simulink model "chris_3R_hsv_all_primitives_sinking_vortex"  (R2024b)
settings: Solver=FixedStepDiscrete  StartTime=0.0  StopTime=30  FixedStep=0.1  MaxStep=0.1  RelTol=1e-3
libraries: neural x110, realtime_pacer_lib x1, simulink x1
(part 6 of 7)

== system chris_3R_hsv_all_primitives_sinking_vortex/tidal_hsv_tuning1/RGB to hue_sat for_celeste/celeste_sat_net/Layer 2/LW{2,1} ==
  "ad{2,1}" : Inport  PortDimensions=6
      mask Display: e = 0.06;c1 = [120 230 180]/255;c2 = ([120 230 180]+0)/(256+128);c3 = ([120 230 180]+128)/(256+128);patch([0 1 1 0],[0 0 1 1],c1);patch([0 1 1 1-e 1-e 0+e],[0 0 1 1-e 0+e 0+e],c2);patch([0 0 1 1-e 0+e 0+e],[0 1 1 1-e 1-e 0+e],c3);plot([0 1 1 0 0],[0 0 1 1 0]);
  "IW{2,1}(1,:)'" : Constant  Value=[1.2757889938032482834984193686977960169315338134765625;-0.7126078429664080005068171885795891284942626953125;-2.413344046511821883171933222911320626735687255859375;-1.458997927672031291734811020432971417903900146484375;-0.83989823818357633999909239719272591173648834228515625;1.7854337780265587820593964352156035602092742919921875]
      mask Display: e = 0.06;c1 = [120 150 230]/255;c2 = ([120 150 230]+0)/383;c3 = ([120 150 230]+128)/383;patch([0 1 1 0],[0 0 1 1],c1);patch([0 1 1 1-e 1-e 0+e],[0 0 1 1-e 0+e 0+e],c2);patch([0 0 1 1-e 0+e 0+e],[0 1 1 1-e 1-e 0+e],c3);plot([0 1 1 0 0],[0 0 1 1 0]);disp('weights');
  "IW{2,1}(2,:)'" : Constant  Value=[-1.6571971168098029725257447353214956820011138916015625;-0.67977626560509663011799830201198346912860870361328125;0.51865396369048488711683830842957831919193267822265625;0.243374659103428425677151381023577414453029632568359375;-0.076285515094898281862612066106521524488925933837890625;1.29330601294184877048110138275660574436187744140625]
      mask Display: e = 0.06;c1 = [120 150 230]/255;c2 = ([120 150 230]+0)/383;c3 = ([120 150 230]+128)/383;patch([0 1 1 0],[0 0 1 1],c1);patch([0 1 1 1-e 1-e 0+e],[0 0 1 1-e 0+e 0+e],c2);patch([0 0 1 1-e 0+e 0+e],[0 1 1 1-e 1-e 0+e],c3);plot([0 1 1 0 0],[0 0 1 1 0]);disp('weights');
  "IW{2,1}(3,:)'" : Constant  Value=[1.377295451076403054457841790281236171722412109375;0.01268764281998376909632586517773233936168253421783447265625;0.0289104963224421605827441084102247259579598903656005859375;-1.145112921630900615355130867101252079010009765625;-1.1470518023551152797523400295176543295383453369140625;0.7180170108229269043675913053448311984539031982421875]
      mask Display: e = 0.06;c1 = [120 150 230]/255;c2 = ([120 150 230]+0)/383;c3 = ([120 150 230]+128)/383;patch([0 1 1 0],[0 0 1 1],c1);patch([0 1 1 1-e 1-e 0+e],[0 0 1 1-e 0+e 0+e],c2);patch([0 0 1 1-e 0+e 0+e],[0 1 1 1-e 1-e 0+e],c3);plot([0 1 1 0 0],[0 0 1 1 0]);disp('weights');
  "IW{2,1}(4,:)'" : Constant  Value=[-0.50505648910016531782929405380855314433574676513671875;1.641889229081123335873826363240368664264678955078125;0.36309788129570963466363764382549561560153961181640625;2.063260495572241115525002896902151405811309814453125;-1.3457901837695616098500295265694148838520050048828125;3.00694287438520913013917379430495202541351318359375]
      mask Display: e = 0.06;c1 = [120 150 230]/255;c2 = ([120 150 230]+0)/383;c3 = ([120 150 230]+128)/383;patch([0 1 1 0],[0 0 1 1],c1);patch([0 1 1 1-e 1-e 0+e],[0 0 1 1-e 0+e 0+e],c2);patch([0 0 1 1-e 0+e 0+e],[0 1 1 1-e 1-e 0+e],c3);plot([0 1 1 0 0],[0 0 1 1 0]);disp('weights');
  "IW{2,1}(5,:)'" : Constant  Value=[1.747547092995427764350324650877155363559722900390625;1.21424683147417855622052229591645300388336181640625;-2.265290257368467674581324899918399751186370849609375;-0.38255863058397288067880026574130170047283172607421875;1.7408214945567326292774623652803711593151092529296875;-1.030400253471217109080271256971172988414764404296875]
      mask Display: e = 0.06;c1 = [120 150 230]/255;c2 = ([120 150 230]+0)/383;c3 = ([120 150 230]+128)/383;patch([0 1 1 0],[0 0 1 1],c1);patch([0 1 1 1-e 1-e 0+e],[0 0 1 1-e 0+e 0+e],c2);patch([0 0 1 1-e 0+e 0+e],[0 1 1 1-e 1-e 0+e],c3);plot([0 1 1 0 0],[0 0 1 1 0]);disp('weights');
  Mux : Mux  Inputs=5
      mask Display: e = 0.06;c1 = [120 150 230]/255;c2 = ([120 150 230]+0)/383;c3 = ([120 150 230]+128)/383;patch([0 1 1 0],[0 0 1 1],c1);patch([0 1 1 1-e 1-e 0+e],[0 0 1 1-e 0+e 0+e],c2);patch([0 0 1 1-e 0+e 0+e],[0 1 1 1-e 1-e 0+e],c3);plot([0 1 1 0 0],[0 0 1 1 0]);disp('Mux');
  dotprod{1..5} (5 alike) : neural/Weight Functions/dotprod
  "lz{2,1}" : Outport
      mask Display: e = 0.06;c1 = [120 230 180]/255;c2 = ([120 230 180]+0)/(256+128);c3 = ([120 230 180]+128)/(256+128);patch([0 1 1 0],[0 0 1 1],c1);patch([0 1 1 1-e 1-e 0+e],[0 0 1 1-e 0+e 0+e],c2);patch([0 0 1 1-e 0+e 0+e],[0 1 1 1-e 1-e 0+e],c3);plot([0 1 1 0 0],[0 0 1 1 0]);
  wires:
  "IW{2,1}(1,:)'"/1 -> dotprod1/1
  "ad{2,1}"/1 -> dotprod1/2, dotprod2/2, dotprod3/2, dotprod4/2, dotprod5/2
  dotprod1/1 -> Mux/1
  "IW{2,1}(2,:)'"/1 -> dotprod2/1
  dotprod2/1 -> Mux/2
  "IW{2,1}(3,:)'"/1 -> dotprod3/1
  dotprod3/1 -> Mux/3
  "IW{2,1}(4,:)'"/1 -> dotprod4/1
  dotprod4/1 -> Mux/4
  "IW{2,1}(5,:)'"/1 -> dotprod5/1
  dotprod5/1 -> Mux/5
  Mux/1 -> "lz{2,1}"/1

== system chris_3R_hsv_all_primitives_sinking_vortex/tidal_hsv_tuning1/RGB to hue_sat for_celeste/celeste_sat_net/Layer 3/Delays 1 ==
  "p{3}" : Inport  PortDimensions=5
      mask Display: e = 0.06;c1 = [120 230 180]/255;c2 = ([120 230 180]+0)/(256+128);c3 = ([120 230 180]+128)/(256+128);patch([0 1 1 0],[0 0 1 1],c1);patch([0 1 1 1-e 1-e 0+e],[0 0 1 1-e 0+e 0+e],c2);patch([0 0 1 1-e 0+e 0+e],[0 1 1 1-e 1-e 0+e],c3);plot([0 1 1 0 0],[0 0 1 1 0]);
  mux : Mux  Inputs=1
      mask Display: e = 0.06;c1 = [120 150 230]/255;c2 = ([120 150 230]+0)/383;c3 = ([120 150 230]+128)/383;patch([0 1 1 0],[0 0 1 1],c1);patch([0 1 1 1-e 1-e 0+e],[0 0 1 1-e 0+e 0+e],c2);patch([0 0 1 1-e 0+e 0+e],[0 1 1 1-e 1-e 0+e],c3);plot([0 1 1 0 0],[0 0 1 1 0]);disp('Mux')
  "pd{3,2}" : Outport
      mask Display: e = 0.06;c1 = [120 230 180]/255;c2 = ([120 230 180]+0)/(256+128);c3 = ([120 230 180]+128)/(256+128);patch([0 1 1 0],[0 0 1 1],c1);patch([0 1 1 1-e 1-e 0+e],[0 0 1 1-e 0+e 0+e],c2);patch([0 0 1 1-e 0+e 0+e],[0 1 1 1-e 1-e 0+e],c3);plot([0 1 1 0 0],[0 0 1 1 0]);
  wires:
  "p{3}"/1 -> mux/1
  mux/1 -> "pd{3,2}"/1

== system chris_3R_hsv_all_primitives_sinking_vortex/tidal_hsv_tuning1/RGB to hue_sat for_celeste/celeste_sat_net/Layer 3/LW{3,2} ==
  "ad{3,2}" : Inport  PortDimensions=5
      mask Display: e = 0.06;c1 = [120 230 180]/255;c2 = ([120 230 180]+0)/(256+128);c3 = ([120 230 180]+128)/(256+128);patch([0 1 1 0],[0 0 1 1],c1);patch([0 1 1 1-e 1-e 0+e],[0 0 1 1-e 0+e 0+e],c2);patch([0 0 1 1-e 0+e 0+e],[0 1 1 1-e 1-e 0+e],c3);plot([0 1 1 0 0],[0 0 1 1 0]);
  "IW{3,2}(1,:)'" : Constant  Value=[-2.69284198651846651273444877006113529205322265625;1.3716092909789459053371274421806447207927703857421875;2.600820941170569167155690593062900006771087646484375;1.14691405759365405714333974174223840236663818359375;-1.59834977518721199629680995712988078594207763671875]
      mask Display: e = 0.06;c1 = [120 150 230]/255;c2 = ([120 150 230]+0)/383;c3 = ([120 150 230]+128)/383;patch([0 1 1 0],[0 0 1 1],c1);patch([0 1 1 1-e 1-e 0+e],[0 0 1 1-e 0+e 0+e],c2);patch([0 0 1 1-e 0+e 0+e],[0 1 1 1-e 1-e 0+e],c3);plot([0 1 1 0 0],[0 0 1 1 0]);disp('weights');
  Mux : Mux  Inputs=1
      mask Display: e = 0.06;c1 = [120 150 230]/255;c2 = ([120 150 230]+0)/383;c3 = ([120 150 230]+128)/383;patch([0 1 1 0],[0 0 1 1],c1);patch([0 1 1 1-e 1-e 0+e],[0 0 1 1-e 0+e 0+e],c2);patch([0 0 1 1-e 0+e 0+e],[0 1 1 1-e 1-e 0+e],c3);plot([0 1 1 0 0],[0 0 1 1 0]);disp('Mux');
  dotprod1 : neural/Weight Functions/dotprod
  "lz{3,2}" : Outport
      mask Display: e = 0.06;c1 = [120 230 180]/255;c2 = ([120 230 180]+0)/(256+128);c3 = ([120 230 180]+128)/(256+128);patch([0 1 1 0],[0 0 1 1],c1);patch([0 1 1 1-e 1-e 0+e],[0 0 1 1-e 0+e 0+e],c2);patch([0 0 1 1-e 0+e 0+e],[0 1 1 1-e 1-e 0+e],c3);plot([0 1 1 0 0],[0 0 1 1 0]);
  wires:
  "IW{3,2}(1,:)'"/1 -> dotprod1/1
  "ad{3,2}"/1 -> dotprod1/2
  dotprod1/1 -> Mux/1
  Mux/1 -> "lz{3,2}"/1

== matlab function chris_3R_hsv_all_primitives_sinking_vortex/Cluster_Controller_HSV_average_direction_and_mag_follower/Cluster Velocities to Cartesian Velocities ==
  data: fwdkin input; xc_err input; x1 output; zc_err input; thC_err input; a_err input; b_err input; C_err input; z1 output; th1 output; x2 output; z2 output; th2 output; x3 output; z3 output; th3 output
function [x1, z1,th1, x2,z2,th2, x3,z3, th3] = InverseJabobian(fwdkin, xc_err, zc_err, thC_err, a_err, b_err, C_err)
%% Unpacking the information from fwd_kin
p = fwdkin(1);
q = fwdkin(2);
beta = fwdkin(3);
xc = fwdkin(4);
yc = fwdkin(5);
theta_c = fwdkin(6);
yc_err = zc_err;
theta_c_err = thC_err;
p_err = a_err;
q_err = b_err;
beta_err = C_err;
%% Inverse Kinematics
  % Calculate x1, y1, and theta1 (Equations 12, 13, and 14)
r = sqrt((q + p*cos(beta))^2 + (p*sin(beta))^2);
  
x1 = xc + (1/3)*r*sin(theta_c);
y1 = yc + (1/3)*r*cos(theta_c);
%theta1 = phi1 - theta_c;
% Calculate x2, y2, and theta2 (Equations 15, 16, and 17)
x2 = xc + (1/3)*r*sin(theta_c) - p*sin(beta/2 + theta_c);
y2 = yc + (1/3)*r*cos(theta_c) - p*cos(beta/2 + theta_c);
%theta2 = phi2 - theta_c;
% Calculate x3, y3, and theta3 (Equations 18, 19, and 20)
x3 = xc + (1/3)*r*sin(theta_c) + q*sin(beta/2 - theta_c);
y3 = yc + (1/3)*r*cos(theta_c) - q*cos(beta/2 - theta_c);
%theta3 = phi3 - theta_c;
%% Now to take the partial derivates
% syms p q beta xc yc theta_c p_err q_err beta_err xc_err yc_err theta_c_err
% 
% % Define the equations
% eqs = [
%   xc + (1/3)*(sqrt((q + p*cos(beta))^2 + (p*sin(beta))^2))*sin(theta_c); % x1
%   yc + (1/3)*(sqrt((q + p*cos(beta))^2 + (p*sin(beta))^2))*cos(theta_c); % y1
%   xc + (1/3)*(sqrt((q + p*cos(beta))^2 + (p*sin(beta))^2))*sin(theta_c) - p*sin(beta/2 + theta_c); % x2
%   yc + (1/3)*(sqrt((q + p*cos(beta))^2 + (p*sin(beta))^2))*cos(theta_c) - p*cos(beta/2 + theta_c); % y2
%   xc + (1/3)*(sqrt((q + p*cos(beta))^2 + (p*sin(beta))^2))*sin(theta_c) + q*sin(beta/2 - theta_c); % x3
%   yc + (1/3)*(sqrt((q + p*cos(beta))^2 + (p*sin(beta))^2))*cos(theta_c) - q*cos(beta/2 - theta_c)  % y3
% ];
% 
% % Define the variables for differentiation
% vars = [p, q, beta, xc, yc, theta_c];
% 
% % Define the errors
% errs = [p_err, q_err, beta_err, xc_err, yc_err, theta_c_err];
% 
% % Initialize an array to store the sums (as symbolic)
% sums = sym(zeros(length(eqs), 1));
% 
% % Loop through equations and variables
% for i = 1:length(eqs)
%   for j = 1:length(vars)
%     derivative = diff(eqs(i), vars(j));
%     sums(i) = sums(i) + derivative * errs(j);
%   end
% end
% 
% % Display the results
% disp(simplify(sums(1)))
% disp(simplify(sums(2)))
% disp(simplify(sums(3)))
% disp(simplify(sums(4)))
% disp(simplify(sums(5)))
% disp(simplify(sums(6)))
%% Now to sum it all up
x1 =(3*xc_err*(p^2 + 2*cos(beta)*p*q + q^2)^(1/2) + p*p_err*sin(theta_c) + q*q_err*sin(theta_c) + p^2*theta_c_err*cos(theta_c) + q^2*theta_c_err*cos(theta_c) + p*q_err*cos(beta)*sin(theta_c) + p_err*q*cos(beta)*sin(theta_c) + 2*p*q*theta_c_err*cos(beta)*cos(theta_c) - beta_err*p*q*sin(beta)*sin(theta_c))/(3*(p^2 + 2*cos(beta)*p*q + q^2)^(1/2));
 
z1 = (3*yc_err*(p^2 + 2*cos(beta)*p*q + q^2)^(1/2) + p*p_err*cos(theta_c) + q*q_err*cos(theta_c) - p^2*theta_c_err*sin(theta_c) - q^2*theta_c_err*sin(theta_c) + p*q_err*cos(beta)*cos(theta_c) + p_err*q*cos(beta)*cos(theta_c) - beta_err*p*q*sin(beta)*cos(theta_c) - 2*p*q*theta_c_err*cos(beta)*sin(theta_c))/(3*(p^2 + 2*cos(beta)*p*q + q^2)^(1/2));
 
x2 = xc_err - p_err*(sin(beta/2 + theta_c) - (sin(theta_c)*(p + q*cos(beta)))/(3*(p^2 + 2*cos(beta)*p*q + q^2)^(1/2))) - beta_err*((p*cos(beta/2 + theta_c))/2 + (p*q*sin(beta)*sin(theta_c))/(3*(p^2 + 2*cos(beta)*p*q + q^2)^(1/2))) + theta_c_err*((cos(theta_c)*(p^2 + 2*cos(beta)*p*q + q^2)^(1/2))/3 - p*cos(beta/2 + theta_c)) + (q_err*sin(theta_c)*(q + p*cos(beta)))/(3*(p^2 + 2*cos(beta)*p*q + q^2)^(1/2));
 
z2 = yc_err - p_err*(cos(beta/2 + theta_c) - (cos(theta_c)*(p + q*cos(beta)))/(3*(p^2 + 2*cos(beta)*p*q + q^2)^(1/2))) + beta_err*((p*sin(beta/2 + theta_c))/2 - (p*q*sin(beta)*cos(theta_c))/(3*(p^2 + 2*cos(beta)*p*q + q^2)^(1/2))) - (theta_c_err*sin(theta_c)*(p^2 + 2*cos(beta)*p*q + q^2)^(1/2))/3 + p*theta_c_err*sin(beta/2 + theta_c) + (q_err*cos(theta_c)*(q + p*cos(beta)))/(3*(p^2 + 2*cos(beta)*p*q + q^2)^(1/2));
 
x3 = xc_err + q_err*(sin(beta/2 - theta_c) + (sin(theta_c)*(q + p*cos(beta)))/(3*(p^2 + 2*cos(beta)*p*q + q^2)^(1/2))) + beta_err*((q*cos(beta/2 - theta_c))/2 - (p*q*sin(beta)*sin(theta_c))/(3*(p^2 + 2*cos(beta)*p*q + q^2)^(1/2))) + (theta_c_err*cos(theta_c)*(p^2 + 2*cos(beta)*p*q + q^2)^(1/2))/3 - q*theta_c_err*cos(beta/2 - theta_c) + (p_err*sin(theta_c)*(p + q*cos(beta)))/(3*(p^2 + 2*cos(beta)*p*q + q^2)^(1/2));
 
z3 = yc_err - theta_c_err*(q*sin(beta/2 - theta_c) + (sin(theta_c)*(p^2 + 2*cos(beta)*p*q + q^2)^(1/2))/3) - q_err*(cos(beta/2 - theta_c) - (cos(theta_c)*(q + p*cos(beta)))/(3*(p^2 + 2*cos(beta)*p*q + q^2)^(1/2))) + beta_err*((q*sin(beta/2 - theta_c))/2 - (p*q*sin(beta)*cos(theta_c))/(3*(p^2 + 2*cos(beta)*p*q + q^2)^(1/2))) + (p_err*cos(theta_c)*(p + q*cos(beta)))/(3*(p^2 + 2*cos(beta)*p*q + q^2)^(1/2));
 
th1 = 0;
th2 = 0;
th3 = 0;

== matlab function chris_3R_hsv_all_primitives_sinking_vortex/Cluster_Controller_HSV_average_direction_and_mag_follower/3_robot HSV to vector/average_hue ==
  data: avg_reading output; readings input
function avg_reading = circularAverage(readings)


  x_sum = 0;
  y_sum = 0;

  for i = 1:length(readings)
    angle = 2 * pi * readings(i); % Convert reading to angle in radians
    x_sum = x_sum + cos(angle);
    y_sum = y_sum + sin(angle);
  end

  x_avg = x_sum / length(readings);
  y_avg = y_sum / length(readings);

  avg_angle = atan2(y_avg, x_avg); % Use atan2 for correct quadrant
  avg_reading = mod(avg_angle / (2 * pi), 1); % Convert back to reading, using mod for wrap-around

end

== matlab function chris_3R_hsv_all_primitives_sinking_vortex/tidal_hsv_tuning1/RGB to hue_sat for_celeste/Color to vector/MATLAB Function ==
  data: velocity input; undead output
function undead = deadzone(velocity)

if abs(velocity)<0.05
    undead=sign(velocity)*0.04;
else
    undead=velocity;
end
end

== matlab function chris_3R_hsv_all_primitives_sinking_vortex/tidal_hsv_tuning1/RGB to hue_sat for_celeste/Color to vector/MATLAB Function1 ==
  data: velocity input; undead output
function undead = deadzone(velocity)

if abs(velocity)<0.05
    undead=sign(velocity)*0.04;
else
    undead=velocity;
end
end

== matlab function chris_3R_hsv_all_primitives_sinking_vortex/tidal_hsv_tuning1/RGB to hue_sat for_celeste/RGB to HSV ==
  data: R output; G output; B output; K output; R input; H output; G input; B input; K input; S output; V output
function [R, G, B, K, H, S, V]= data_augmentation(R, G, B, K)

  R = squeeze(R);
  G = squeeze(G); 
  B = squeeze(B);
  K = squeeze(K);
  
   
  % if strcmp(robot_name, "celeste")  % Use strcmp for string comparison
  %   % Normalize RGB to [0, 1]
    R = (R - 141) / 1006;
    G = (G - 237) / 1160;
    B = (B - 241) / 1073;
    K = (K - 868) / 3032;
   
  % elseif strcmp(robot_name, "tidal") % Use strcmp for string comparison
  %   % Normalize RGB to [0, 1]
    % R = (R - 104) / 966;
    % G = (G - 180) / 1183;
    % B = (B - 174) / 1026;
    % K = (K - 678) / 3021;
   
  % elseif strcmp(robot_name, "pacific-blue") % Use strcmp for string comparison 
  % Normalize RGB to [0, 1]
  %  R = (R - 127) / 1012;
  %  G = (G - 218) / 1121;
  %  B = (B - 219) / 971;
  %  K = (K - 842) / 2824;

    R = max(min(R, 1), 0);
    G = max(min(G, 1), 0);
    B = max(min(B, 1), 0);
    K = max(min(K, 1), 0);

    Cmax = max(max(R, G), B);
    Cmin = min(min(R, G), B);
    delta = Cmax - Cmin;

    % Initialize H, S, V as scalar values
    H = 0;
    S = 0;
    V = Cmax;

    % Calculate Hue
    if delta ~= 0
        if Cmax == R
            H = 60 * mod((G - B) / delta, 6);
        elseif Cmax == G
            H = 60 * (((B - R) / delta) + 2);
        elseif Cmax == B
            H = 60 * (((R - G) / delta) + 4);
        end
        H = H / 360;
    end

    % Calculate Saturation
    if Cmax ~= 0
        S = delta / Cmax;
    end

end

== matlab function chris_3R_hsv_all_primitives_sinking_vortex/tidal_hsv_tuning/RGB to hue_sat for tidal/Color to vector/MATLAB Function ==
  data: velocity input; undead output
function undead = deadzone(velocity)

if abs(velocity)<0.05
    undead=sign(velocity)*0.04;
else
    undead=velocity;
end
end

== matlab function chris_3R_hsv_all_primitives_sinking_vortex/tidal_hsv_tuning/RGB to hue_sat for tidal/Color to vector/MATLAB Function1 ==
  data: velocity input; undead output
function undead = deadzone(velocity)

if abs(velocity)<0.05
    undead=sign(velocity)*0.04;
else
    undead=velocity;
end
end

== matlab function chris_3R_hsv_all_primitives_sinking_vortex/tidal_hsv_tuning/RGB to hue_sat for tidal/RGB to HSV ==
  data: R output; G output; B output; K output; R input; H output; G input; B input; K input; S output; V output
function [R, G, B, K, H, S, V]= data_augmentation(R, G, B, K)

  R = squeeze(R);
  G = squeeze(G); 
  B = squeeze(B);
  K = squeeze(K);
  
   
  % if strcmp(robot_name, "celeste")  % Use strcmp for string comparison
  %   % Normalize RGB to [0, 1]
  %   R = (R - 141) / 1006;
  %   G = (G - 237) / 1160;
  %   B = (B - 241) / 1073;
  %   K = (K - 868) / 3032;
   
  % elseif strcmp(robot_name, "tidal") % Use strcmp for string comparison
  %   % Normalize RGB to [0, 1]
    R = (R - 104) / 966;
    G = (G - 180) / 1183;
    B = (B - 174) / 1026;
    K = (K - 678) / 3021;
   
  % elseif strcmp(robot_name, "pacific-blue") % Use strcmp for string comparison 
  % Normalize RGB to [0, 1]
  %  R = (R - 127) / 1012;
  %  G = (G - 218) / 1121;
  %  B = (B - 219) / 971;
  %  K = (K - 842) / 2824;

    R = max(min(R, 1), 0);
    G = max(min(G, 1), 0);
    B = max(min(B, 1), 0);
    K = max(min(K, 1), 0);

    Cmax = max(max(R, G), B);
    Cmin = min(min(R, G), B);
    delta = Cmax - Cmin;

    % Initialize H, S, V as scalar values
    H = 0;
    S = 0;
    V = Cmax;

    % Calculate Hue
    if delta ~= 0
        if Cmax == R
            H = 60 * mod((G - B) / delta, 6);
        elseif Cmax == G
            H = 60 * (((B - R) / delta) + 2);
        elseif Cmax == B
            H = 60 * (((R - G) / delta) + 4);
        end
        H = H / 360;
    end

    % Calculate Saturation
    if Cmax ~= 0
        S = delta / Cmax;
    end

end

== matlab function chris_3R_hsv_all_primitives_sinking_vortex/pacific_blue_hsv_tuning1/RGB to HSV to vel - pacific-blue1/Color to vector/MATLAB Function ==
  data: velocity input; undead output
function undead = deadzone(velocity)

if abs(velocity)<0.05
    undead=sign(velocity)*0.04;
else
    undead=velocity;
end
end

== matlab function chris_3R_hsv_all_primitives_sinking_vortex/Cluster_Controller_HSV_direction_only/3_robot HSV to vector/average_hue ==
  data: avg_reading output; readings input
function avg_reading = circularAverage(readings)


  x_sum = 0;
  y_sum = 0;

  for i = 1:length(readings)
    angle = 2 * pi * readings(i); % Convert reading to angle in radians
    x_sum = x_sum + cos(angle);
    y_sum = y_sum + sin(angle);
  end

  x_avg = x_sum / length(readings);
  y_avg = y_sum / length(readings);

  avg_angle = atan2(y_avg, x_avg); % Use atan2 for correct quadrant
  avg_reading = mod(avg_angle / (2 * pi), 1); % Convert back to reading, using mod for wrap-around

end

== matlab function chris_3R_hsv_all_primitives_sinking_vortex/Cluster_Controller_HSV_direction_only/Cartesian to Cluster Variables ==
  data: fwdkin output; x1 input; x_c output; y1 input; th1 input; x2 input; y2 input; th2 input; x3 input; y3 input; th3 input; y_c output; th_c output; a output; b output; c output
function [fwdkin, x_c, y_c, th_c, a, b, c]   = Forward_Kinematics(x1, y1, th1, x2,y2,th2, x3,y3,th3)
% Centre frame
x_c = (x1+x2+x3)/3;
y_c = (y1+y2+y3)/3;
theta_c = atan2((2/3)*x1 - (1/3)*(x2 + x3), (2/3)*y1 - (1/3)*(y2 + y3));
% SAS Properties of triangle
p = sqrt((x1 - x2)^2 + (y1 - y2)^2);
q = sqrt((x3 - x1)^2 + (y1 - y3)^2);
beta = acos((p^2 + q^2 - (x3 - x2)^2 - (y3 - y2)^2) / (2*p*q));
% Rotation vectors
phi1 = th1 + theta_c;
phi2 = th2 + theta_c;
phi3 = th3 + theta_c;
a =p;
b = q;
c = beta;
th_c = theta_c;
fwdkin = [0 0 0 0 0 0];
fwdkin(1) =a;
fwdkin(2) =b;
fwdkin(3) =c;
fwdkin(4) =x_c;
fwdkin(5) =y_c;
fwdkin(6) =th_c;

== matlab function chris_3R_hsv_all_primitives_sinking_vortex/Cluster_Controller_HSV_magnitude_unsure/3_robot HSV to vector/MATLAB Function ==
  data: x output; x1 input; y output; y1 input; z1 input; x2 input; y2 input; z2 input; x3 input; y3 input; z3 input
function [x, y] = steepestDescent(x1, y1, z1, x2, y2, z2, x3, y3, z3)
  % Create vectors AB and AC
  AB = [x2 - x1, y2 - y1, z2 - z1];
  AC = [x3 - x1, y3 - y1, z3 - z1];

  % Calculate the cross product to get the normal vector
  N = cross(AB, AC);

  % Get the direction of steepest descent (-N)
  descent = -N;

  % Normalize the vector to have unit length in the xy-plane
  magnitude = sqrt(descent(1)^2 + descent(2)^2);
  x = descent(1) / magnitude;
  y = descent(2) / magnitude;
end

== matlab function chris_3R_hsv_all_primitives_sinking_vortex/Cluster_Controller_HSV_magnitude_unsure/Cartesian to Cluster Variables ==
  data: fwdkin output; x1 input; x_c output; y1 input; th1 input; x2 input; y2 input; th2 input; x3 input; y3 input; th3 input; y_c output; th_c output; a output; b output; c output
function [fwdkin, x_c, y_c, th_c, a, b, c]   = Forward_Kinematics(x1, y1, th1, x2,y2,th2, x3,y3,th3)
% Centre frame
x_c = (x1+x2+x3)/3;
y_c = (y1+y2+y3)/3;
theta_c = atan2((2/3)*x1 - (1/3)*(x2 + x3), (2/3)*y1 - (1/3)*(y2 + y3));
% SAS Properties of triangle
p = sqrt((x1 - x2)^2 + (y1 - y2)^2);
q = sqrt((x3 - x1)^2 + (y1 - y3)^2);
beta = acos((p^2 + q^2 - (x3 - x2)^2 - (y3 - y2)^2) / (2*p*q));
% Rotation vectors
phi1 = th1 + theta_c;
phi2 = th2 + theta_c;
phi3 = th3 + theta_c;
a =p;
b = q;
c = beta;
th_c = theta_c;
fwdkin = [0 0 0 0 0 0];
fwdkin(1) =a;
fwdkin(2) =b;
fwdkin(3) =c;
fwdkin(4) =x_c;
fwdkin(5) =y_c;
fwdkin(6) =th_c;

== matlab function chris_3R_hsv_all_primitives_sinking_vortex/Robot_signal_processing_2/Global to Body Rotation Matrix ==
  data: u input; y output
function y = fcn(u)

y = [cos(u) -sin(u) 0; sin(u) cos(u) 0; 0 0 1];

== matlab function chris_3R_hsv_all_primitives_sinking_vortex/Cluster_Controller_HSV_magnitude_unsure/Cluster Velocities to Cartesian Velocities ==
  data: fwdkin input; xc_err input; x1 output; zc_err input; thC_err input; a_err input; b_err input; C_err input; z1 output; th1 output; x2 output; z2 output; th2 output; x3 output; z3 output; th3 output
function [x1, z1,th1, x2,z2,th2, x3,z3, th3] = InverseJabobian(fwdkin, xc_err, zc_err, thC_err, a_err, b_err, C_err)
%% Unpacking the information from fwd_kin
p = fwdkin(1);
q = fwdkin(2);
beta = fwdkin(3);
xc = fwdkin(4);
yc = fwdkin(5);
theta_c = fwdkin(6);
yc_err = zc_err;
theta_c_err = thC_err;
p_err = a_err;
q_err = b_err;
beta_err = C_err;
%% Inverse Kinematics
  % Calculate x1, y1, and theta1 (Equations 12, 13, and 14)
r = sqrt((q + p*cos(beta))^2 + (p*sin(beta))^2);
  
x1 = xc + (1/3)*r*sin(theta_c);
y1 = yc + (1/3)*r*cos(theta_c);
%theta1 = phi1 - theta_c;
% Calculate x2, y2, and theta2 (Equations 15, 16, and 17)
x2 = xc + (1/3)*r*sin(theta_c) - p*sin(beta/2 + theta_c);
y2 = yc + (1/3)*r*cos(theta_c) - p*cos(beta/2 + theta_c);
%theta2 = phi2 - theta_c;
% Calculate x3, y3, and theta3 (Equations 18, 19, and 20)
x3 = xc + (1/3)*r*sin(theta_c) + q*sin(beta/2 - theta_c);
y3 = yc + (1/3)*r*cos(theta_c) - q*cos(beta/2 - theta_c);
%theta3 = phi3 - theta_c;
%% Now to take the partial derivates
% syms p q beta xc yc theta_c p_err q_err beta_err xc_err yc_err theta_c_err
% 
% % Define the equations
% eqs = [
%   xc + (1/3)*(sqrt((q + p*cos(beta))^2 + (p*sin(beta))^2))*sin(theta_c); % x1
%   yc + (1/3)*(sqrt((q + p*cos(beta))^2 + (p*sin(beta))^2))*cos(theta_c); % y1
%   xc + (1/3)*(sqrt((q + p*cos(beta))^2 + (p*sin(beta))^2))*sin(theta_c) - p*sin(beta/2 + theta_c); % x2
%   yc + (1/3)*(sqrt((q + p*cos(beta))^2 + (p*sin(beta))^2))*cos(theta_c) - p*cos(beta/2 + theta_c); % y2
%   xc + (1/3)*(sqrt((q + p*cos(beta))^2 + (p*sin(beta))^2))*sin(theta_c) + q*sin(beta/2 - theta_c); % x3
%   yc + (1/3)*(sqrt((q + p*cos(beta))^2 + (p*sin(beta))^2))*cos(theta_c) - q*cos(beta/2 - theta_c)  % y3
% ];
% 
% % Define the variables for differentiation
% vars = [p, q, beta, xc, yc, theta_c];
% 
% % Define the errors
% errs = [p_err, q_err, beta_err, xc_err, yc_err, theta_c_err];
% 
% % Initialize an array to store the sums (as symbolic)
% sums = sym(zeros(length(eqs), 1));
% 
% % Loop through equations and variables
% for i = 1:length(eqs)
%   for j = 1:length(vars)
%     derivative = diff(eqs(i), vars(j));
%     sums(i) = sums(i) + derivative * errs(j);
%   end
% end
% 
% % Display the results
% disp(simplify(sums(1)))
% disp(simplify(sums(2)))
% disp(simplify(sums(3)))
% disp(simplify(sums(4)))
% disp(simplify(sums(5)))
% disp(simplify(sums(6)))
%% Now to sum it all up
x1 =(3*xc_err*(p^2 + 2*cos(beta)*p*q + q^2)^(1/2) + p*p_err*sin(theta_c) + q*q_err*sin(theta_c) + p^2*theta_c_err*cos(theta_c) + q^2*theta_c_err*cos(theta_c) + p*q_err*cos(beta)*sin(theta_c) + p_err*q*cos(beta)*sin(theta_c) + 2*p*q*theta_c_err*cos(beta)*cos(theta_c) - beta_err*p*q*sin(beta)*sin(theta_c))/(3*(p^2 + 2*cos(beta)*p*q + q^2)^(1/2));
 
z1 = (3*yc_err*(p^2 + 2*cos(beta)*p*q + q^2)^(1/2) + p*p_err*cos(theta_c) + q*q_err*cos(theta_c) - p^2*theta_c_err*sin(theta_c) - q^2*theta_c_err*sin(theta_c) + p*q_err*cos(beta)*cos(theta_c) + p_err*q*cos(beta)*cos(theta_c) - beta_err*p*q*sin(beta)*cos(theta_c) - 2*p*q*theta_c_err*cos(beta)*sin(theta_c))/(3*(p^2 + 2*cos(beta)*p*q + q^2)^(1/2));
 
x2 = xc_err - p_err*(sin(beta/2 + theta_c) - (sin(theta_c)*(p + q*cos(beta)))/(3*(p^2 + 2*cos(beta)*p*q + q^2)^(1/2))) - beta_err*((p*cos(beta/2 + theta_c))/2 + (p*q*sin(beta)*sin(theta_c))/(3*(p^2 + 2*cos(beta)*p*q + q^2)^(1/2))) + theta_c_err*((cos(theta_c)*(p^2 + 2*cos(beta)*p*q + q^2)^(1/2))/3 - p*cos(beta/2 + theta_c)) + (q_err*sin(theta_c)*(q + p*cos(beta)))/(3*(p^2 + 2*cos(beta)*p*q + q^2)^(1/2));
 
z2 = yc_err - p_err*(cos(beta/2 + theta_c) - (cos(theta_c)*(p + q*cos(beta)))/(3*(p^2 + 2*cos(beta)*p*q + q^2)^(1/2))) + beta_err*((p*sin(beta/2 + theta_c))/2 - (p*q*sin(beta)*cos(theta_c))/(3*(p^2 + 2*cos(beta)*p*q + q^2)^(1/2))) - (theta_c_err*sin(theta_c)*(p^2 + 2*cos(beta)*p*q + q^2)^(1/2))/3 + p*theta_c_err*sin(beta/2 + theta_c) + (q_err*cos(theta_c)*(q + p*cos(beta)))/(3*(p^2 + 2*cos(beta)*p*q + q^2)^(1/2));
 
x3 = xc_err + q_err*(sin(beta/2 - theta_c) + (sin(theta_c)*(q + p*cos(beta)))/(3*(p^2 + 2*cos(beta)*p*q + q^2)^(1/2))) + beta_err*((q*cos(beta/2 - theta_c))/2 - (p*q*sin(beta)*sin(theta_c))/(3*(p^2 + 2*cos(beta)*p*q + q^2)^(1/2))) + (theta_c_err*cos(theta_c)*(p^2 + 2*cos(beta)*p*q + q^2)^(1/2))/3 - q*theta_c_err*cos(beta/2 - theta_c) + (p_err*sin(theta_c)*(p + q*cos(beta)))/(3*(p^2 + 2*cos(beta)*p*q + q^2)^(1/2));
 
z3 = yc_err - theta_c_err*(q*sin(beta/2 - theta_c) + (sin(theta_c)*(p^2 + 2*cos(beta)*p*q + q^2)^(1/2))/3) - q_err*(cos(beta/2 - theta_c) - (cos(theta_c)*(q + p*cos(beta)))/(3*(p^2 + 2*cos(beta)*p*q + q^2)^(1/2))) + beta_err*((q*sin(beta/2 - theta_c))/2 - (p*q*sin(beta)*cos(theta_c))/(3*(p^2 + 2*cos(beta)*p*q + q^2)^(1/2))) + (p_err*cos(theta_c)*(p + q*cos(beta)))/(3*(p^2 + 2*cos(beta)*p*q + q^2)^(1/2));
 
th1 = 0;
th2 = 0;
th3 = 0;

== matlab function chris_3R_hsv_all_primitives_sinking_vortex/tidal_hsv_tuning/RGB to hue_sat for tidal/hue_post_processor ==
  data: hue output; hue_nn_sin input; hue_nn_cos input
function hue = hue_post_processing(hue_nn_sin, hue_nn_cos)

hue_nn_sin = (hue_nn_sin+1)/2;
hue_nn_cos = (hue_nn_cos+1)/2;

hue = atan2(hue_nn_sin, hue_nn_cos);
hue(hue < 0) = hue(hue < 0) + 2 * pi;
hue = hue / (2 * pi);


hue = max(0,min(hue,1));
end

== matlab function chris_3R_hsv_all_primitives_sinking_vortex/tidal_hsv_tuning/RGB to hue_sat for tidal/sat_post_processor ==
  data: sat output; sat_nn_output input
function sat = sat_post_processing(sat_nn_output)

sat = (sat_nn_output+1)/2;

sat = max(0,min(sat,1));
end

== matlab function chris_3R_hsv_all_primitives_sinking_vortex/tidal_hsv_tuning1/RGB to hue_sat for_celeste/hue_post_processor ==
  data: hue output; hue_nn_sin input; hue_nn_cos input
function hue = hue_post_processing(hue_nn_sin, hue_nn_cos)

hue_nn_sin = (hue_nn_sin+1)/2;
hue_nn_cos = (hue_nn_cos+1)/2;

hue = atan2(hue_nn_sin, hue_nn_cos);
hue(hue < 0) = hue(hue < 0) + 2 * pi;
hue = hue / (2 * pi);


hue = max(0,min(hue,1));
end

== matlab function chris_3R_hsv_all_primitives_sinking_vortex/tidal_hsv_tuning1/RGB to hue_sat for_celeste/sat_post_processor ==
  data: sat output; sat_nn_output input
function sat = sat_post_processing(sat_nn_output)

sat = (sat_nn_output+1)/2;

sat = max(0,min(sat,1));
end

== matlab function chris_3R_hsv_all_primitives_sinking_vortex/tidal_hsv_tuning1/RGB to hue_sat for_celeste/sat_pre_processor1 ==
  data: data output; data_raw input
function data = data_normalizing(data_raw)

data = (data_raw*2)-1;


end

== matlab function chris_3R_hsv_all_primitives_sinking_vortex/tidal_hsv_tuning/RGB to hue_sat for tidal/sat_pre_processor1 ==
  data: data output; data_raw input
function data = data_normalizing(data_raw)

data = (data_raw*2)-1;


end

== matlab function chris_3R_hsv_all_primitives_sinking_vortex/pacific_blue_hsv_tuning1/RGB to HSV to vel - pacific-blue1/Color to vector/MATLAB Function1 ==
  data: velocity input; undead output
function undead = deadzone(velocity)

if abs(velocity)<0.05
    undead=sign(velocity)*0.04;
else
    undead=velocity;
end
end

== matlab function chris_3R_hsv_all_primitives_sinking_vortex/Robot_signal_processing_3/Global to Body Rotation Matrix ==
  data: u input; y output
function y = fcn(u)

y = [cos(u) -sin(u) 0; sin(u) cos(u) 0; 0 0 1];

== matlab function chris_3R_hsv_all_primitives_sinking_vortex/pacific_blue_hsv_tuning1/RGB to HSV to vel - pacific-blue1/RGB to HSV ==
  data: R output; G output; B output; K output; R input; H output; G input; B input; K input; S output; V output
function [R, G, B, K, H, S, V]= data_augmentation(R, G, B, K)

  R = squeeze(R);
  G = squeeze(G); 
  B = squeeze(B);
  K = squeeze(K);
  
   
  % if strcmp(robot_name, "celeste")  % Use strcmp for string comparison
  %   % Normalize RGB to [0, 1]
  %   R = (R - 141) / 1006;
  %   G = (G - 237) / 1160;
  %   B = (B - 241) / 1073;
  %   K = (K - 868) / 3032;
   
  % elseif strcmp(robot_name, "tidal") % Use strcmp for string comparison
  %   % Normalize RGB to [0, 1]
  %   R = (R - 104) / 966;
  %   G = (G - 180) / 1183;
  %   B = (B - 174) / 1026;
  %   K = (K - 678) / 3021;
   
  % elseif strcmp(robot_name, "pacific-blue") % Use strcmp for string comparison 
  % Normalize RGB to [0, 1]
    R = (R - 127) / 1012;
    G = (G - 218) / 1121;
    B = (B - 219) / 971;
    K = (K - 842) / 2824;

    R = max(min(R, 1), 0);
    G = max(min(G, 1), 0);
    B = max(min(B, 1), 0);
    K = max(min(K, 1), 0);

    Cmax = max(max(R, G), B);
    Cmin = min(min(R, G), B);
    delta = Cmax - Cmin;

    % Initialize H, S, V as scalar values
    H = 0;
    S = 0;
    V = Cmax;

    % Calculate Hue
    if delta ~= 0
        if Cmax == R
            H = 60 * mod((G - B) / delta, 6);
        elseif Cmax == G
            H = 60 * (((B - R) / delta) + 2);
        elseif Cmax == B
            H = 60 * (((R - G) / delta) + 4);
        end
        H = H / 360;
    end

    % Calculate Saturation
    if Cmax ~= 0
        S = delta / Cmax;
    end

end

== matlab function chris_3R_hsv_all_primitives_sinking_vortex/pacific_blue_hsv_tuning1/RGB to HSV to vel - pacific-blue1/hue_post_processor ==
  data: hue output; hue_nn_sin input; hue_nn_cos input
function hue = hue_post_processing(hue_nn_sin, hue_nn_cos)

hue_nn_sin = (hue_nn_sin+1)/2;
hue_nn_cos = (hue_nn_cos+1)/2;

hue = atan2(hue_nn_sin, hue_nn_cos);
hue(hue < 0) = hue(hue < 0) + 2 * pi;
hue = hue / (2 * pi);


hue = max(0,min(hue,1));
end

== matlab function chris_3R_hsv_all_primitives_sinking_vortex/pacific_blue_hsv_tuning1/RGB to HSV to vel - pacific-blue1/sat_post_processor ==
  data: sat output; sat_nn_output input
function sat = sat_post_processing(sat_nn_output)

sat = (sat_nn_output+1)/2;

sat = max(0,min(sat,1));
end

== matlab function chris_3R_hsv_all_primitives_sinking_vortex/pacific_blue_hsv_tuning1/RGB to HSV to vel - pacific-blue1/sat_post_processor1 ==
  data: data output; data_raw input
function data = data_normalizing(data_raw)

data = (data_raw*2)-1;


end

== matlab function chris_3R_hsv_all_primitives_sinking_vortex/Cluster_Controller_HSV_direction_only/Cluster Velocities to Cartesian Velocities ==
  data: fwdkin input; xc_err input; x1 output; zc_err input; thC_err input; a_err input; b_err input; C_err input; z1 output; th1 output; x2 output; z2 output; th2 output; x3 output; z3 output; th3 output
function [x1, z1,th1, x2,z2,th2, x3,z3, th3] = InverseJabobian(fwdkin, xc_err, zc_err, thC_err, a_err, b_err, C_err)
%% Unpacking the information from fwd_kin
p = fwdkin(1);
q = fwdkin(2);
beta = fwdkin(3);
xc = fwdkin(4);
yc = fwdkin(5);
theta_c = fwdkin(6);
yc_err = zc_err;
theta_c_err = thC_err;
p_err = a_err;
q_err = b_err;
beta_err = C_err;
%% Inverse Kinematics
  % Calculate x1, y1, and theta1 (Equations 12, 13, and 14)
r = sqrt((q + p*cos(beta))^2 + (p*sin(beta))^2);
  
x1 = xc + (1/3)*r*sin(theta_c);
y1 = yc + (1/3)*r*cos(theta_c);
%theta1 = phi1 - theta_c;
% Calculate x2, y2, and theta2 (Equations 15, 16, and 17)
x2 = xc + (1/3)*r*sin(theta_c) - p*sin(beta/2 + theta_c);
y2 = yc + (1/3)*r*cos(theta_c) - p*cos(beta/2 + theta_c);
%theta2 = phi2 - theta_c;
% Calculate x3, y3, and theta3 (Equations 18, 19, and 20)
x3 = xc + (1/3)*r*sin(theta_c) + q*sin(beta/2 - theta_c);
y3 = yc + (1/3)*r*cos(theta_c) - q*cos(beta/2 - theta_c);
%theta3 = phi3 - theta_c;
%% Now to take the partial derivates
% syms p q beta xc yc theta_c p_err q_err beta_err xc_err yc_err theta_c_err
% 
% % Define the equations
% eqs = [
%   xc + (1/3)*(sqrt((q + p*cos(beta))^2 + (p*sin(beta))^2))*sin(theta_c); % x1
%   yc + (1/3)*(sqrt((q + p*cos(beta))^2 + (p*sin(beta))^2))*cos(theta_c); % y1
%   xc + (1/3)*(sqrt((q + p*cos(beta))^2 + (p*sin(beta))^2))*sin(theta_c) - p*sin(beta/2 + theta_c); % x2
%   yc + (1/3)*(sqrt((q + p*cos(beta))^2 + (p*sin(beta))^2))*cos(theta_c) - p*cos(beta/2 + theta_c); % y2
%   xc + (1/3)*(sqrt((q + p*cos(beta))^2 + (p*sin(beta))^2))*sin(theta_c) + q*sin(beta/2 - theta_c); % x3
%   yc + (1/3)*(sqrt((q + p*cos(beta))^2 + (p*sin(beta))^2))*cos(theta_c) - q*cos(beta/2 - theta_c)  % y3
% ];
% 
% % Define the variables for differentiation
% vars = [p, q, beta, xc, yc, theta_c];
% 
% % Define the errors
% errs = [p_err, q_err, beta_err, xc_err, yc_err, theta_c_err];
% 
% % Initialize an array to store the sums (as symbolic)
% sums = sym(zeros(length(eqs), 1));
% 
% % Loop through equations and variables
% for i = 1:length(eqs)
%   for j = 1:length(vars)
%     derivative = diff(eqs(i), vars(j));
%     sums(i) = sums(i) + derivative * errs(j);
%   end
% end
% 
% % Display the results
% disp(simplify(sums(1)))
% disp(simplify(sums(2)))
% disp(simplify(sums(3)))
% disp(simplify(sums(4)))
% disp(simplify(sums(5)))
% disp(simplify(sums(6)))
%% Now to sum it all up
x1 =(3*xc_err*(p^2 + 2*cos(beta)*p*q + q^2)^(1/2) + p*p_err*sin(theta_c) + q*q_err*sin(theta_c) + p^2*theta_c_err*cos(theta_c) + q^2*theta_c_err*cos(theta_c) + p*q_err*cos(beta)*sin(theta_c) + p_err*q*cos(beta)*sin(theta_c) + 2*p*q*theta_c_err*cos(beta)*cos(theta_c) - beta_err*p*q*sin(beta)*sin(theta_c))/(3*(p^2 + 2*cos(beta)*p*q + q^2)^(1/2));
 
z1 = (3*yc_err*(p^2 + 2*cos(beta)*p*q + q^2)^(1/2) + p*p_err*cos(theta_c) + q*q_err*cos(theta_c) - p^2*theta_c_err*sin(theta_c) - q^2*theta_c_err*sin(theta_c) + p*q_err*cos(beta)*cos(theta_c) + p_err*q*cos(beta)*cos(theta_c) - beta_err*p*q*sin(beta)*cos(theta_c) - 2*p*q*theta_c_err*cos(beta)*sin(theta_c))/(3*(p^2 + 2*cos(beta)*p*q + q^2)^(1/2));
 
x2 = xc_err - p_err*(sin(beta/2 + theta_c) - (sin(theta_c)*(p + q*cos(beta)))/(3*(p^2 + 2*cos(beta)*p*q + q^2)^(1/2))) - beta_err*((p*cos(beta/2 + theta_c))/2 + (p*q*sin(beta)*sin(theta_c))/(3*(p^2 + 2*cos(beta)*p*q + q^2)^(1/2))) + theta_c_err*((cos(theta_c)*(p^2 + 2*cos(beta)*p*q + q^2)^(1/2))/3 - p*cos(beta/2 + theta_c)) + (q_err*sin(theta_c)*(q + p*cos(beta)))/(3*(p^2 + 2*cos(beta)*p*q + q^2)^(1/2));
 
z2 = yc_err - p_err*(cos(beta/2 + theta_c) - (cos(theta_c)*(p + q*cos(beta)))/(3*(p^2 + 2*cos(beta)*p*q + q^2)^(1/2))) + beta_err*((p*sin(beta/2 + theta_c))/2 - (p*q*sin(beta)*cos(theta_c))/(3*(p^2 + 2*cos(beta)*p*q + q^2)^(1/2))) - (theta_c_err*sin(theta_c)*(p^2 + 2*cos(beta)*p*q + q^2)^(1/2))/3 + p*theta_c_err*sin(beta/2 + theta_c) + (q_err*cos(theta_c)*(q + p*cos(beta)))/(3*(p^2 + 2*cos(beta)*p*q + q^2)^(1/2));
 
x3 = xc_err + q_err*(sin(beta/2 - theta_c) + (sin(theta_c)*(q + p*cos(beta)))/(3*(p^2 + 2*cos(beta)*p*q + q^2)^(1/2))) + beta_err*((q*cos(beta/2 - theta_c))/2 - (p*q*sin(beta)*sin(theta_c))/(3*(p^2 + 2*cos(beta)*p*q + q^2)^(1/2))) + (theta_c_err*cos(theta_c)*(p^2 + 2*cos(beta)*p*q + q^2)^(1/2))/3 - q*theta_c_err*cos(beta/2 - theta_c) + (p_err*sin(theta_c)*(p + q*cos(beta)))/(3*(p^2 + 2*cos(beta)*p*q + q^2)^(1/2));
 
z3 = yc_err - theta_c_err*(q*sin(beta/2 - theta_c) + (sin(theta_c)*(p^2 + 2*cos(beta)*p*q + q^2)^(1/2))/3) - q_err*(cos(beta/2 - theta_c) - (cos(theta_c)*(q + p*cos(beta)))/(3*(p^2 + 2*cos(beta)*p*q + q^2)^(1/2))) + beta_err*((q*sin(beta/2 - theta_c))/2 - (p*q*sin(beta)*cos(theta_c))/(3*(p^2 + 2*cos(beta)*p*q + q^2)^(1/2))) + (p_err*cos(theta_c)*(p + q*cos(beta)))/(3*(p^2 + 2*cos(beta)*p*q + q^2)^(1/2));
 
th1 = 0;
th2 = 0;
th3 = 0;

== matlab function chris_3R_hsv_all_primitives_sinking_vortex/Cluster_Controller_HSV_steepest_descent/3_robot HSV to vector/MATLAB Function ==
  data: x output; x1 input; y output; y1 input; z1 input; x2 input; y2 input; z2 input; x3 input; y3 input; z3 input
function [x, y] = steepestDescent(x1, y1, z1, x2, y2, z2, x3, y3, z3)
  % Create vectors AB and AC
  AB = [x2 - x1, y2 - y1, z2 - z1];
  AC = [x3 - x1, y3 - y1, z3 - z1];

  % Calculate the cross product to get the normal vector
  N = cross(-AB, AC);

  % Get the direction of steepest descent (-N)
  descent =-N;

  % Normalize the vector to have unit length in the xy-plane
  magnitude = sqrt(descent(1)^2 + descent(2)^2);
  x = descent(1) / magnitude;
  y = descent(2) / magnitude;
  x = -x/10;
  y = -y/10;
end

== matlab function chris_3R_hsv_all_primitives_sinking_vortex/Cluster_Controller_setpoint/Cartesian to Cluster Variables ==
  data: fwdkin output; x1 input; x_c output; y1 input; th1 input; x2 input; y2 input; th2 input; x3 input; y3 input; th3 input; y_c output; th_c output; a output; b output; c output
function [fwdkin, x_c, y_c, th_c, a, b, c]   = Forward_Kinematics(x1, y1, th1, x2,y2,th2, x3,y3,th3)
% Centre frame
x_c = (x1+x2+x3)/3;
y_c = (y1+y2+y3)/3;
theta_c = atan2((2/3)*x1 - (1/3)*(x2 + x3), (2/3)*y1 - (1/3)*(y2 + y3));
% SAS Properties of triangle
p = sqrt((x1 - x2)^2 + (y1 - y2)^2);
q = sqrt((x3 - x1)^2 + (y1 - y3)^2);
beta = acos((p^2 + q^2 - (x3 - x2)^2 - (y3 - y2)^2) / (2*p*q));
% Rotation vectors
phi1 = th1 + theta_c;
phi2 = th2 + theta_c;
phi3 = th3 + theta_c;
a =p;
b = q;
c = beta;
th_c = theta_c;
fwdkin = [0 0 0 0 0 0];
fwdkin(1) =a;
fwdkin(2) =b;
fwdkin(3) =c;
fwdkin(4) =x_c;
fwdkin(5) =y_c;
fwdkin(6) =th_c;

== matlab function chris_3R_hsv_all_primitives_sinking_vortex/Cluster_Controller_HSV_steepest_descent/Cartesian to Cluster Variables ==
  data: fwdkin output; x1 input; x_c output; y1 input; th1 input; x2 input; y2 input; th2 input; x3 input; y3 input; th3 input; y_c output; th_c output; a output; b output; c output; phi1 output; phi2 output; phi3 output
function [fwdkin, x_c, y_c, th_c, a, b, c,phi1,phi2,phi3]   = Forward_Kinematics(x1, y1, th1, x2,y2,th2, x3,y3,th3)
% Centre frame
x_c = (x1+x2+x3)/3;
y_c = (y1+y2+y3)/3;
theta_c = atan2((2/3)*x1 - (1/3)*(x2 + x3), (2/3)*y1 - (1/3)*(y2 + y3));
% SAS Properties of triangle
p = sqrt((x1 - x2)^2 + (y1 - y2)^2);
q = sqrt((x3 - x1)^2 + (y1 - y3)^2);
beta = acos((p^2 + q^2 - (x3 - x2)^2 - (y3 - y2)^2) / (2*p*q));
% Rotation vectors
phi1 = th1 + theta_c;
phi2 = th2 + theta_c;
phi3 = th3 + theta_c;
a =p;
b = q;
c = beta;
th_c = theta_c;
fwdkin = [0 0 0 0 0 0];
fwdkin(1) =a;
fwdkin(2) =b;
fwdkin(3) =c;
fwdkin(4) =x_c;
fwdkin(5) =y_c;
fwdkin(6) =th_c;

== matlab function chris_3R_hsv_all_primitives_sinking_vortex/Cluster_Controller_HSV_steepest_descent/Cluster Velocities to Cartesian Velocities ==
  data: fwdkin input; xc_err input; x1 output; zc_err input; thC_err input; a_err input; b_err input; C_err input; z1 output; th1 output; x2 output; z2 output; th2 output; x3 output; z3 output; th3 output
function [x1, z1,th1, x2,z2,th2, x3,z3, th3] = InverseJabobian(fwdkin, xc_err, zc_err, thC_err, a_err, b_err, C_err)
%% Unpacking the information from fwd_kin
p = fwdkin(1);
q = fwdkin(2);
beta = fwdkin(3);
xc = fwdkin(4);
yc = fwdkin(5);
theta_c = fwdkin(6);
yc_err = zc_err;
theta_c_err = thC_err;
p_err = a_err;
q_err = b_err;
beta_err = C_err;
%% Inverse Kinematics
  % Calculate x1, y1, and theta1 (Equations 12, 13, and 14)
r = sqrt((q + p*cos(beta))^2 + (p*sin(beta))^2);
  
x1 = xc + (1/3)*r*sin(theta_c);
y1 = yc + (1/3)*r*cos(theta_c);
%theta1 = phi1 - theta_c;
% Calculate x2, y2, and theta2 (Equations 15, 16, and 17)
x2 = xc + (1/3)*r*sin(theta_c) - p*sin(beta/2 + theta_c);
y2 = yc + (1/3)*r*cos(theta_c) - p*cos(beta/2 + theta_c);
%theta2 = phi2 - theta_c;
% Calculate x3, y3, and theta3 (Equations 18, 19, and 20)
x3 = xc + (1/3)*r*sin(theta_c) + q*sin(beta/2 - theta_c);
y3 = yc + (1/3)*r*cos(theta_c) - q*cos(beta/2 - theta_c);
%theta3 = phi3 - theta_c;
%% Now to take the partial derivates
% syms p q beta xc yc theta_c p_err q_err beta_err xc_err yc_err theta_c_err
% 
% % Define the equations
% eqs = [
%   xc + (1/3)*(sqrt((q + p*cos(beta))^2 + (p*sin(beta))^2))*sin(theta_c); % x1
%   yc + (1/3)*(sqrt((q + p*cos(beta))^2 + (p*sin(beta))^2))*cos(theta_c); % y1
%   xc + (1/3)*(sqrt((q + p*cos(beta))^2 + (p*sin(beta))^2))*sin(theta_c) - p*sin(beta/2 + theta_c); % x2
%   yc + (1/3)*(sqrt((q + p*cos(beta))^2 + (p*sin(beta))^2))*cos(theta_c) - p*cos(beta/2 + theta_c); % y2
%   xc + (1/3)*(sqrt((q + p*cos(beta))^2 + (p*sin(beta))^2))*sin(theta_c) + q*sin(beta/2 - theta_c); % x3
%   yc + (1/3)*(sqrt((q + p*cos(beta))^2 + (p*sin(beta))^2))*cos(theta_c) - q*cos(beta/2 - theta_c)  % y3
% ];
% 
% % Define the variables for differentiation
% vars = [p, q, beta, xc, yc, theta_c];
% 
% % Define the errors
% errs = [p_err, q_err, beta_err, xc_err, yc_err, theta_c_err];
% 
% % Initialize an array to store the sums (as symbolic)
% sums = sym(zeros(length(eqs), 1));
% 
% % Loop through equations and variables
% for i = 1:length(eqs)
%   for j = 1:length(vars)
%     derivative = diff(eqs(i), vars(j));
%     sums(i) = sums(i) + derivative * errs(j);
%   end
% end
% 
% % Display the results
% disp(simplify(sums(1)))
% disp(simplify(sums(2)))
% disp(simplify(sums(3)))
% disp(simplify(sums(4)))
% disp(simplify(sums(5)))
% disp(simplify(sums(6)))
%% Now to sum it all up
x1 =(3*xc_err*(p^2 + 2*cos(beta)*p*q + q^2)^(1/2) + p*p_err*sin(theta_c) + q*q_err*sin(theta_c) + p^2*theta_c_err*cos(theta_c) + q^2*theta_c_err*cos(theta_c) + p*q_err*cos(beta)*sin(theta_c) + p_err*q*cos(beta)*sin(theta_c) + 2*p*q*theta_c_err*cos(beta)*cos(theta_c) - beta_err*p*q*sin(beta)*sin(theta_c))/(3*(p^2 + 2*cos(beta)*p*q + q^2)^(1/2));
 
z1 = (3*yc_err*(p^2 + 2*cos(beta)*p*q + q^2)^(1/2) + p*p_err*cos(theta_c) + q*q_err*cos(theta_c) - p^2*theta_c_err*sin(theta_c) - q^2*theta_c_err*sin(theta_c) + p*q_err*cos(beta)*cos(theta_c) + p_err*q*cos(beta)*cos(theta_c) - beta_err*p*q*sin(beta)*cos(theta_c) - 2*p*q*theta_c_err*cos(beta)*sin(theta_c))/(3*(p^2 + 2*cos(beta)*p*q + q^2)^(1/2));
 
x2 = xc_err - p_err*(sin(beta/2 + theta_c) - (sin(theta_c)*(p + q*cos(beta)))/(3*(p^2 + 2*cos(beta)*p*q + q^2)^(1/2))) - beta_err*((p*cos(beta/2 + theta_c))/2 + (p*q*sin(beta)*sin(theta_c))/(3*(p^2 + 2*cos(beta)*p*q + q^2)^(1/2))) + theta_c_err*((cos(theta_c)*(p^2 + 2*cos(beta)*p*q + q^2)^(1/2))/3 - p*cos(beta/2 + theta_c)) + (q_err*sin(theta_c)*(q + p*cos(beta)))/(3*(p^2 + 2*cos(beta)*p*q + q^2)^(1/2));
 
z2 = yc_err - p_err*(cos(beta/2 + theta_c) - (cos(theta_c)*(p + q*cos(beta)))/(3*(p^2 + 2*cos(beta)*p*q + q^2)^(1/2))) + beta_err*((p*sin(beta/2 + theta_c))/2 - (p*q*sin(beta)*cos(theta_c))/(3*(p^2 + 2*cos(beta)*p*q + q^2)^(1/2))) - (theta_c_err*sin(theta_c)*(p^2 + 2*cos(beta)*p*q + q^2)^(1/2))/3 + p*theta_c_err*sin(beta/2 + theta_c) + (q_err*cos(theta_c)*(q + p*cos(beta)))/(3*(p^2 + 2*cos(beta)*p*q + q^2)^(1/2));
 
x3 = xc_err + q_err*(sin(beta/2 - theta_c) + (sin(theta_c)*(q + p*cos(beta)))/(3*(p^2 + 2*cos(beta)*p*q + q^2)^(1/2))) + beta_err*((q*cos(beta/2 - theta_c))/2 - (p*q*sin(beta)*sin(theta_c))/(3*(p^2 + 2*cos(beta)*p*q + q^2)^(1/2))) + (theta_c_err*cos(theta_c)*(p^2 + 2*cos(beta)*p*q + q^2)^(1/2))/3 - q*theta_c_err*cos(beta/2 - theta_c) + (p_err*sin(theta_c)*(p + q*cos(beta)))/(3*(p^2 + 2*cos(beta)*p*q + q^2)^(1/2));
 
z3 = yc_err - theta_c_err*(q*sin(beta/2 - theta_c) + (sin(theta_c)*(p^2 + 2*cos(beta)*p*q + q^2)^(1/2))/3) - q_err*(cos(beta/2 - theta_c) - (cos(theta_c)*(q + p*cos(beta)))/(3*(p^2 + 2*cos(beta)*p*q + q^2)^(1/2))) + beta_err*((q*sin(beta/2 - theta_c))/2 - (p*q*sin(beta)*cos(theta_c))/(3*(p^2 + 2*cos(beta)*p*q + q^2)^(1/2))) + (p_err*cos(theta_c)*(p + q*cos(beta)))/(3*(p^2 + 2*cos(beta)*p*q + q^2)^(1/2));
 
th1 = 0;
th2 = 0;
th3 = 0;
